simulink model "RAC"  (R2022b)
settings: Solver=FixedStepAuto  StartTime=0.0  StopTime=50000000  FixedStep=1  RelTol=1e-3
libraries: simulink x50
(part 1 of 2)
settings Model: Creator=sadamu  LastModifiedBy=程一帆
settings OptimizationCC: DefaultParameterBehavior=Inlined  BufferReuse=off  GlobalBufferReuse=off  ExpressionFolding=off  EnableMemcpy=off  PassReuseOutputArgsAs=Individual arguments  NoFixptDivByZeroProtection=on  EfficientFloat2IntCast=on  OptimizeDataStoreBuffers=off  BusAssignmentInplaceUpdate=off  OptimizationLevel=level0  EfficientTunableParamExpr=on
settings DebuggingCC: ParameterTunabilityLossMsg=error  AllowSymbolicDim=off
settings SFSimCC: MATLABDynamicMemAlloc=off
settings RTWCC: Description=Embedded Coder  SystemTargetFile=ert.tlc  GenCodeOnly=on  TemplateMakefile=ert_default_tmf
settings CodeAppCC: GenerateComments=off  IgnoreCustomStorageClasses=off  OperatorAnnotations=on  SimulinkDataObjDesc=on  SFDataObjDesc=on  SimulinkBlockComments=off
settings ERTTargetCC: TargetLangStandard=C99 (ISO)  GenerateSampleERTMain=on  CodeInterfacePackaging=Reusable function  InlinedParameterPlacement=NonHierarchical  ERTCustomFileTemplate=example_file_process.tlc
settings ConfigComp: CovMetricSettings=dcmwe  DVMaxProcessTime=3600  DVTestSuiteOptimization=Auto  DVDetectOutOfBounds=on  DVModelReferenceHarness=on

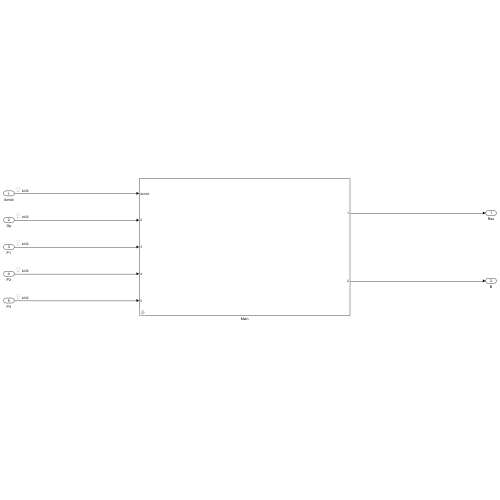
[thumbnail: Simulink's stored preview of the top-level diagram]
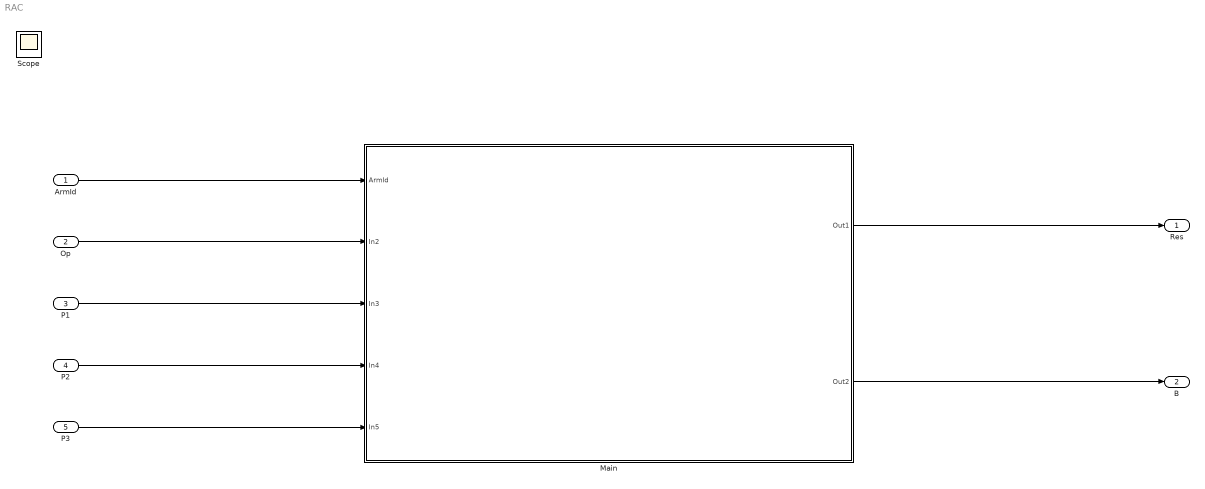
== system RAC ==
  ArmId : Inport  OutDataTypeStr=int32
  Op : Inport  Port=2  OutDataTypeStr=int32
  P1 : Inport  Port=3  OutDataTypeStr=int32
  P2 : Inport  Port=4  OutDataTypeStr=int32
  P3 : Inport  Port=5  OutDataTypeStr=int32
  Main : Subsystem  mask{POOL_SIZE=16}
      mask DialogControl ParameterGroupVar Prompt: 参数
  Res : Outport
  B : Outport  Port=2
  Scope : Scope
  wires:
  ArmId/1 -> Main/1(ArmId)
  Op/1 -> Main/2(In2)
  P1/1 -> Main/3(In3)
  P2/1 -> Main/4(In4)
  P3/1 -> Main/5(In5)
  Main/1(Out1) -> Res/1
  Main/2(Out2) -> B/1

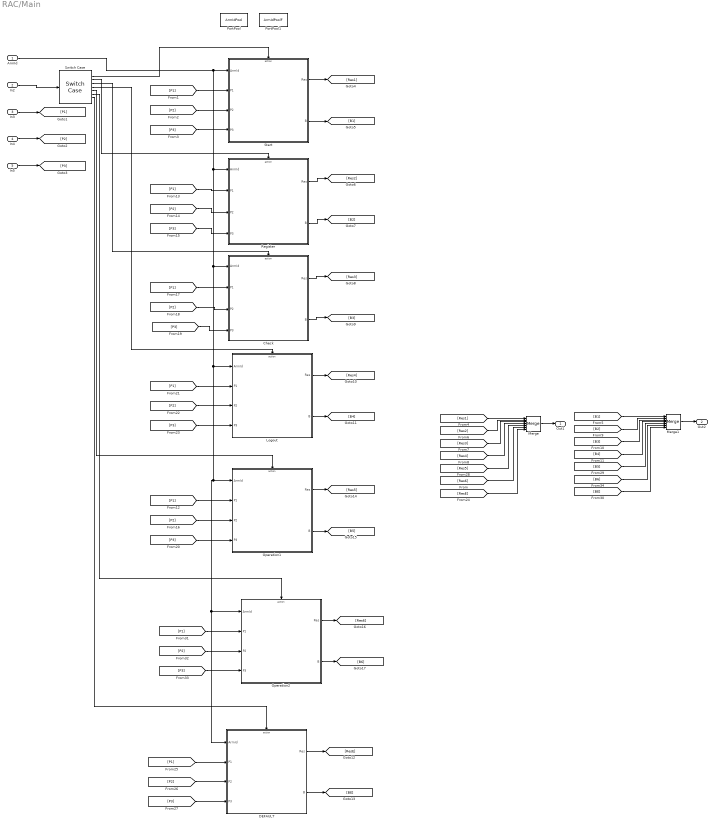
== system RAC/Main ==
  ArmId : Inport
  In2 : Inport  Port=2
  In3 : Inport  Port=3
  In4 : Inport  Port=4
  In5 : Inport  Port=5
  Check : Subsystem  TreatAsAtomicUnit=on
  DEFAULT : Subsystem  TreatAsAtomicUnit=on
  Logout : Subsystem  TreatAsAtomicUnit=on
  Merge : Merge  Inputs=7
  Merge1 : Merge  Inputs=7
  Operation1 : Subsystem  TreatAsAtomicUnit=on
  Operation2 : Subsystem  TreatAsAtomicUnit=on
  PortPool : DataStoreMemory  DataStoreName=ArmIdPool  WriteAfterWriteMsg=warning  ShowAdditionalParam=off  OutDataTypeStr=int32  Dimensions=POOL_SIZE
  PortPool1 : DataStoreMemory  DataStoreName=ArmIdPoolF  WriteAfterWriteMsg=warning  ShowAdditionalParam=off  OutDataTypeStr=int32  Dimensions=POOL_SIZE
  Register : Subsystem  TreatAsAtomicUnit=on
  Start : Subsystem  TreatAsAtomicUnit=on
  Switch Case : SwitchCase  CaseConditions={10001, 10002, 10004, 10008, 10016, 10032}
  Out1 : Outport
  Out2 : Outport  Port=2
  wires:
  DEFAULT/1(Res) -> [ResE]
  Start/1(Res) -> [Res1]
  In2/1 -> Switch Case/1
  [P3] -> Logout/4(P3)
  Check/1(Res) -> [Res3]
  [B4] -> Merge1/4
  [Res1] -> Merge/1
  [B1] -> Merge1/1
  Logout/2(B) -> [B4]
  Check/2(B) -> [B3]
  Start/2(B) -> [B1]
  [Res3] -> Merge/3
  [P3] -> Register/4(P3)
  [P1] -> Start/2(P1)
  [Res5] -> Merge/5
  [Res2] -> Merge/2
  [Res4] -> Merge/4
  [P2] -> Register/3(P2)
  [B2] -> Merge1/2
  [P3] -> DEFAULT/4(P3)
  Register/1(Res) -> [Res2]
  [P1] -> Register/2(P1)
  [P2] -> Start/3(P2)
  [B3] -> Merge1/3
  [P2] -> DEFAULT/3(P2)
  Switch Case/2 -> Register/Action
  In4/1 -> [P2]
  Switch Case/7 -> DEFAULT/Action
  Register/2(B) -> [B2]
  Switch Case/4 -> Logout/Action
  [P2] -> Check/3(P2)
  [B5] -> Merge1/5
  In5/1 -> [P3]
  [P3] -> Start/4(P3)
  [P1] -> DEFAULT/2(P1)
  [P2] -> Logout/3(P2)
  DEFAULT/2(B) -> [BE]
  Switch Case/3 -> Check/Action
  [P1] -> Check/2(P1)
  [P3] -> Check/4(P3)
  Logout/1(Res) -> [Res4]
  Switch Case/1 -> Start/Action
  Merge1/1 -> Out2/1
  [P1] -> Logout/2(P1)
  In3/1 -> [P1]
  Merge/1 -> Out1/1
  [P1] -> Operation1/2(P1)
  [P2] -> Operation1/3(P2)
  Operation1/1(Res) -> [Res5]
  Operation1/2(B) -> [B5]
  [P3] -> Operation1/4(P3)
  Switch Case/5 -> Operation1/Action
  Operation2/1(Res) -> [Res6]
  [P1] -> Operation2/2(P1)
  Operation2/2(B) -> [B6]
  [P3] -> Operation2/4(P3)
  ArmId/1 -> Operation1/1(ArmId), Operation2/1(ArmId), DEFAULT/1(ArmId), Logout/1(ArmId), Check/1(ArmId), Register/1(ArmId), Start/1(ArmId)
  [P2] -> Operation2/3(P2)
  Switch Case/6 -> Operation2/Action
  [B6] -> Merge1/6
  [BE] -> Merge1/7
  [Res6] -> Merge/6
  [ResE] -> Merge/7

== system RAC/Main/Check ==
  ArmId : Inport
  P1 : Inport  Port=2
  P2 : Inport  Port=3
  P3 : Inport  Port=4
  Action Port : ActionPort  ActionPortLabel=case [ 10004 ]:
  Compare To Constant : simulink/Logic and Bit Operations/Compare To Constant  relop===  const=0  OutDataTypeStr=boolean
  Error : Subsystem  TreatAsAtomicUnit=on
  Handle : Subsystem  TreatAsAtomicUnit=on
  If : If  IfExpression=u1 ~= 0
  Merge : Merge
  Merge1 : Merge
  Res : Outport
  B : Outport  Port=2
  wires:
  P1/1 -> Handle/2(P1)
  P2/1 -> Handle/3(P2)
  P3/1 -> Handle/4(P3)
  Merge/1 -> Res/1
  Error/2(B) -> Merge1/1
  If/1 -> Error/Action
  If/2 -> Handle/Action
  Merge1/1 -> B/1
  ArmId/1 -> Handle/1(ArmId), Compare To Constant/1
  Error/1(Res) -> Merge/1
  Handle/2(B) -> Merge1/2
  Handle/1(Res) -> Merge/2
  Compare To Constant/1 -> If/1

== system RAC/Main/DEFAULT ==
  ArmId : Inport
  P1 : Inport  Port=2
  P2 : Inport  Port=3
  P3 : Inport  Port=4
  Action Port : ActionPort  ActionPortLabel=default:
  Constant : Constant  Value=-2  OutDataTypeStr=int32
  Constant1 : Constant  Value=0  OutDataTypeStr=int32
  Terminator{,1..3} (4 alike) : Terminator
  Res : Outport
  B : Outport  Port=2
  wires:
  Constant/1 -> Res/1
  ArmId/1 -> Terminator/1
  P1/1 -> Terminator1/1
  P2/1 -> Terminator2/1
  P3/1 -> Terminator3/1
  Constant1/1 -> B/1

== system RAC/Main/Logout ==
  ArmId : Inport
  P1 : Inport  Port=2
  P2 : Inport  Port=3
  P3 : Inport  Port=4
  Action Port : ActionPort  ActionPortLabel=case [ 10008 ]:
  Compare To Constant : simulink/Logic and Bit Operations/Compare To Constant  relop===  const=0  OutDataTypeStr=boolean
  Error : Subsystem  TreatAsAtomicUnit=on
  Handle : Subsystem  TreatAsAtomicUnit=on
  If : If  IfExpression=u1 ~= 0
  Merge : Merge
  Merge1 : Merge
  Res : Outport
  B : Outport  Port=2
  wires:
  ArmId/1 -> Handle/1(ArmId), Compare To Constant/1
  Compare To Constant/1 -> If/1
  P2/1 -> Handle/3(P2)
  Error/2(B) -> Merge1/1
  P1/1 -> Handle/2(P1)
  Handle/1(Res) -> Merge/2
  Merge1/1 -> B/1
  Error/1(Res) -> Merge/1
  Merge/1 -> Res/1
  If/1 -> Error/Action
  If/2 -> Handle/Action
  P3/1 -> Handle/4(P3)
  Handle/2(B) -> Merge1/2

== system RAC/Main/Operation1 ==
  ArmId : Inport
  P1 : Inport  Port=2
  P2 : Inport  Port=3
  P3 : Inport  Port=4
  Action Port : ActionPort  ActionPortLabel=case [ 10016 ]:
  Compare To Constant : simulink/Logic and Bit Operations/Compare To Constant  relop===  const=0  OutDataTypeStr=boolean
  Error : Subsystem  TreatAsAtomicUnit=on
  Handle : Subsystem  TreatAsAtomicUnit=on
  If : If  IfExpression=u1 ~= 0
  Merge : Merge
  Merge1 : Merge
  Res : Outport
  B : Outport  Port=2
  wires:
  ArmId/1 -> Handle/1(ArmId), Compare To Constant/1
  Compare To Constant/1 -> If/1
  P2/1 -> Handle/3(P2)
  Error/2(B) -> Merge1/1
  P1/1 -> Handle/2(P1)
  Handle/1(Res) -> Merge/2
  Merge1/1 -> B/1
  Error/1(Res) -> Merge/1
  Merge/1 -> Res/1
  If/1 -> Error/Action
  If/2 -> Handle/Action
  P3/1 -> Handle/4(P3)
  Handle/2(B) -> Merge1/2

== system RAC/Main/Operation2 ==
  ArmId : Inport
  P1 : Inport  Port=2
  P2 : Inport  Port=3
  P3 : Inport  Port=4
  Action Port : ActionPort  ActionPortLabel=case [ 10032 ]:
  Compare To Constant : simulink/Logic and Bit Operations/Compare To Constant  relop===  const=0  OutDataTypeStr=boolean
  Error : Subsystem  TreatAsAtomicUnit=on
  Handle : Subsystem  TreatAsAtomicUnit=on
  If : If  IfExpression=u1 ~= 0
  Merge : Merge
  Merge1 : Merge
  Res : Outport
  B : Outport  Port=2
  wires:
  ArmId/1 -> Handle/1(ArmId), Compare To Constant/1
  Compare To Constant/1 -> If/1
  P2/1 -> Handle/3(P2)
  Error/2(B) -> Merge1/1
  P1/1 -> Handle/2(P1)
  Handle/1(Res) -> Merge/2
  Merge1/1 -> B/1
  Error/1(Res) -> Merge/1
  Merge/1 -> Res/1
  If/1 -> Error/Action
  If/2 -> Handle/Action
  P3/1 -> Handle/4(P3)
  Handle/2(B) -> Merge1/2

== system RAC/Main/Register ==
  ArmId : Inport
  P1 : Inport  Port=2
  P2 : Inport  Port=3
  P3 : Inport  Port=4
  Action Port : ActionPort  ActionPortLabel=case [ 10002 ]:
  Compare To Constant : simulink/Logic and Bit Operations/Compare To Constant  relop===  const=0  OutDataTypeStr=boolean
  Error : Subsystem  TreatAsAtomicUnit=on
  Handle : Subsystem  TreatAsAtomicUnit=on
  If : If  IfExpression=u1 ~= 0
  Merge : Merge
  Merge1 : Merge
  Res : Outport
  B : Outport  Port=2
  wires:
  P1/1 -> Handle/2(P1)
  P2/1 -> Handle/3(P2)
  P3/1 -> Handle/4(P3)
  Merge/1 -> Res/1
  Error/2(B) -> Merge1/1
  If/1 -> Error/Action
  If/2 -> Handle/Action
  Merge1/1 -> B/1
  ArmId/1 -> Handle/1(ArmId), Compare To Constant/1
  Error/1(Res) -> Merge/1
  Handle/2(B) -> Merge1/2
  Handle/1(Res) -> Merge/2
  Compare To Constant/1 -> If/1

== system RAC/Main/Start ==
  ArmId : Inport
  P1 : Inport  Port=2
  P2 : Inport  Port=3
  P3 : Inport  Port=4
  Action Port : ActionPort  ActionPortLabel=case [ 10001 ]:
  Compare To Constant : simulink/Logic and Bit Operations/Compare To Constant  relop===  const=0  OutDataTypeStr=boolean
  Error : Subsystem  TreatAsAtomicUnit=on
  Handle : Subsystem  TreatAsAtomicUnit=on
  If : If  IfExpression=u1 ~= 0
  Merge : Merge
  Merge1 : Merge
  Res : Outport
  B : Outport  Port=2
  wires:
  ArmId/1 -> Handle/1(ArmId), Compare To Constant/1
  Compare To Constant/1 -> If/1
  If/1 -> Error/Action
  If/2 -> Handle/Action
  Error/1(Res) -> Merge/1
  Handle/1(Res) -> Merge/2
  Merge/1 -> Res/1
  Merge1/1 -> B/1
  Error/2(B) -> Merge1/1
  Handle/2(B) -> Merge1/2
  P1/1 -> Handle/2(P1)
  P2/1 -> Handle/3(P2)
  P3/1 -> Handle/4(P3)

== system RAC/Main/Check/Error ==
  Action Port : ActionPort  ActionPortLabel=if(u1 ~= 0)
  Constant : Constant  Value=-1  OutDataTypeStr=int32
  Constant1 : Constant  Value=0  OutDataTypeStr=int32
  Res : Outport
  B : Outport  Port=2
  wires:
  Constant/1 -> Res/1
  Constant1/1 -> B/1

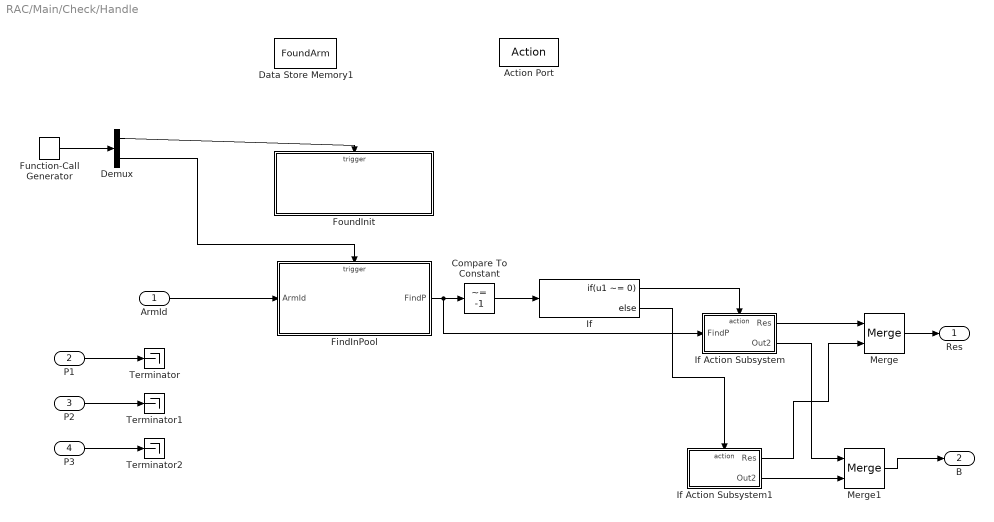
== system RAC/Main/Check/Handle ==
  ArmId : Inport
  P1 : Inport  Port=2
  P2 : Inport  Port=3
  P3 : Inport  Port=4
  Action Port : ActionPort  ActionPortLabel=else
  Compare To Constant : simulink/Logic and Bit Operations/Compare To Constant  relop=~=  const=-1  OutDataTypeStr=boolean
  Data Store Memory1 : DataStoreMemory  DataStoreName=FoundArm  WriteAfterWriteMsg=warning  InitialValue=-1  ShowAdditionalParam=off  OutDataTypeStr=int32
  Demux : Demux  Outputs=2
  FindInPool : Subsystem
  FoundInit : Subsystem
  Function-Call Generator : simulink/Ports & Subsystems/Function-Call Generator  sample_time=1  numberOfIterations=1  DisallowWideOutput=off
  If : If  IfExpression=u1 ~= 0
  If Action Subsystem : Subsystem  TreatAsAtomicUnit=on
  If Action Subsystem1 : Subsystem  TreatAsAtomicUnit=on
  Merge : Merge
  Merge1 : Merge
  Terminator : Terminator
  Terminator1 : Terminator
  Terminator2 : Terminator
  Res : Outport
  B : Outport  Port=2
  wires:
  Function-Call Generator/1 -> Demux/1
  Demux/1 -> FoundInit/Trigger
  Demux/2 -> FindInPool/Trigger
  ArmId/1 -> FindInPool/1(ArmId)
  P1/1 -> Terminator/1
  P2/1 -> Terminator1/1
  P3/1 -> Terminator2/1
  FindInPool/1(FindP) -> If Action Subsystem/1(FindP), Compare To Constant/1
  Compare To Constant/1 -> If/1
  If/1 -> If Action Subsystem/Action
  Merge/1 -> Res/1
  Merge1/1 -> B/1
  If Action Subsystem/1(Res) -> Merge/1
  If Action Subsystem/2(Out2) -> Merge1/1
  If Action Subsystem1/1(Res) -> Merge/2
  If Action Subsystem1/2(Out2) -> Merge1/2
  If/2 -> If Action Subsystem1/Action

== system RAC/Main/Logout/Error ==
  Action Port : ActionPort  ActionPortLabel=if(u1 ~= 0)
  Constant : Constant  Value=-1  OutDataTypeStr=int32
  Constant1 : Constant  Value=0  OutDataTypeStr=int32
  Res : Outport
  B : Outport  Port=2
  wires:
  Constant/1 -> Res/1
  Constant1/1 -> B/1

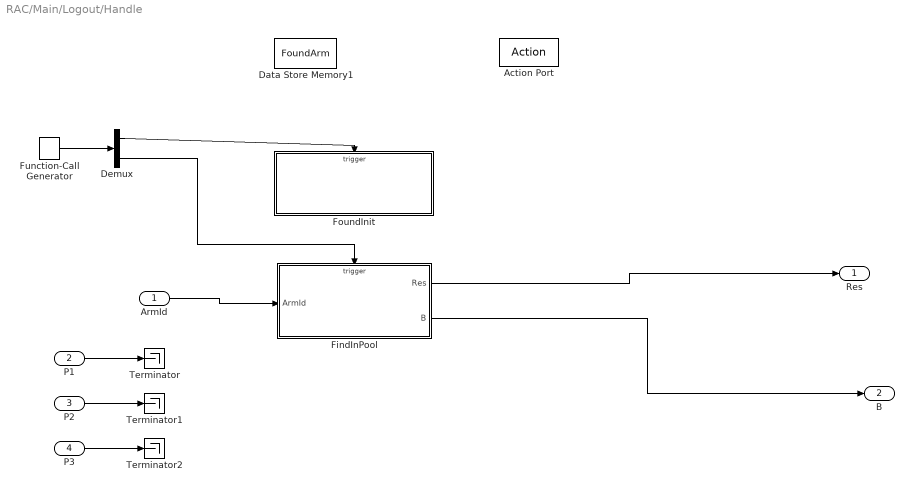
== system RAC/Main/Logout/Handle ==
  ArmId : Inport
  P1 : Inport  Port=2
  P2 : Inport  Port=3
  P3 : Inport  Port=4
  Action Port : ActionPort  ActionPortLabel=else
  Data Store Memory1 : DataStoreMemory  DataStoreName=FoundArm  WriteAfterWriteMsg=warning  InitialValue=-1  ShowAdditionalParam=off  OutDataTypeStr=int32
  Demux : Demux  Outputs=2
  FindInPool : Subsystem
  FoundInit : Subsystem
  Function-Call Generator : simulink/Ports & Subsystems/Function-Call Generator  sample_time=1  numberOfIterations=1  DisallowWideOutput=off
  Terminator : Terminator
  Terminator1 : Terminator
  Terminator2 : Terminator
  Res : Outport
  B : Outport  Port=2
  wires:
  Function-Call Generator/1 -> Demux/1
  Demux/1 -> FoundInit/Trigger
  Demux/2 -> FindInPool/Trigger
  ArmId/1 -> FindInPool/1(ArmId)
  P1/1 -> Terminator/1
  P2/1 -> Terminator1/1
  P3/1 -> Terminator2/1
  FindInPool/1(Res) -> Res/1
  FindInPool/2(B) -> B/1

== system RAC/Main/Operation1/Error ==
  Action Port : ActionPort  ActionPortLabel=if(u1 ~= 0)
  Constant : Constant  Value=-1  OutDataTypeStr=int32
  Constant1 : Constant  Value=0  OutDataTypeStr=int32
  Res : Outport
  B : Outport  Port=2
  wires:
  Constant/1 -> Res/1
  Constant1/1 -> B/1

== system RAC/Main/Operation1/Handle ==
  ArmId : Inport
  P1 : Inport  Port=2
  P2 : Inport  Port=3
  P3 : Inport  Port=4
  Action Port : ActionPort  ActionPortLabel=else
  Data Store Memory1 : DataStoreMemory  DataStoreName=FoundArm  WriteAfterWriteMsg=warning  InitialValue=-1  ShowAdditionalParam=off  OutDataTypeStr=int32
  Demux : Demux  Outputs=2
  FindInPool : Subsystem
  FoundInit : Subsystem
  Function-Call Generator : simulink/Ports & Subsystems/Function-Call Generator  sample_time=1  numberOfIterations=1  DisallowWideOutput=off
  Res : Outport
  B : Outport  Port=2
  wires:
  Function-Call Generator/1 -> Demux/1
  Demux/1 -> FoundInit/Trigger
  Demux/2 -> FindInPool/Trigger
  ArmId/1 -> FindInPool/1(ArmId)
  P1/1 -> FindInPool/2(P1)
  P2/1 -> FindInPool/3(P2)
  P3/1 -> FindInPool/4(P3)
  FindInPool/1(Res) -> Res/1
  FindInPool/2(B) -> B/1

== system RAC/Main/Operation2/Error ==
  Action Port : ActionPort
  Constant : Constant  Value=-1  OutDataTypeStr=int32
  Constant1 : Constant  Value=0  OutDataTypeStr=int32
  Res : Outport
  B : Outport  Port=2
  wires:
  Constant/1 -> Res/1
  Constant1/1 -> B/1

== system RAC/Main/Operation2/Handle ==
  ArmId : Inport
  P1 : Inport  Port=2
  P2 : Inport  Port=3
  P3 : Inport  Port=4
  Action Port : ActionPort
  Data Store Memory1 : DataStoreMemory  DataStoreName=FoundArm  WriteAfterWriteMsg=warning  InitialValue=-1  ShowAdditionalParam=off  OutDataTypeStr=int32
  Demux : Demux  Outputs=2
  FindInPool : Subsystem
  FoundInit : Subsystem
  Function-Call Generator : simulink/Ports & Subsystems/Function-Call Generator  sample_time=1  numberOfIterations=1  DisallowWideOutput=off
  Res : Outport
  B : Outport  Port=2
  wires:
  Function-Call Generator/1 -> Demux/1
  Demux/1 -> FoundInit/Trigger
  Demux/2 -> FindInPool/Trigger
  ArmId/1 -> FindInPool/1(ArmId)
  P1/1 -> FindInPool/2(P1)
  P2/1 -> FindInPool/3(P2)
  P3/1 -> FindInPool/4(P3)
  FindInPool/1(Res) -> Res/1
  FindInPool/2(B) -> B/1

== system RAC/Main/Register/Error ==
  Action Port : ActionPort  ActionPortLabel=if(u1 ~= 0)
  Constant : Constant  Value=-1  OutDataTypeStr=int32
  Constant1 : Constant  Value=0  OutDataTypeStr=int32
  Res : Outport
  B : Outport  Port=2
  wires:
  Constant/1 -> Res/1
  Constant1/1 -> B/1

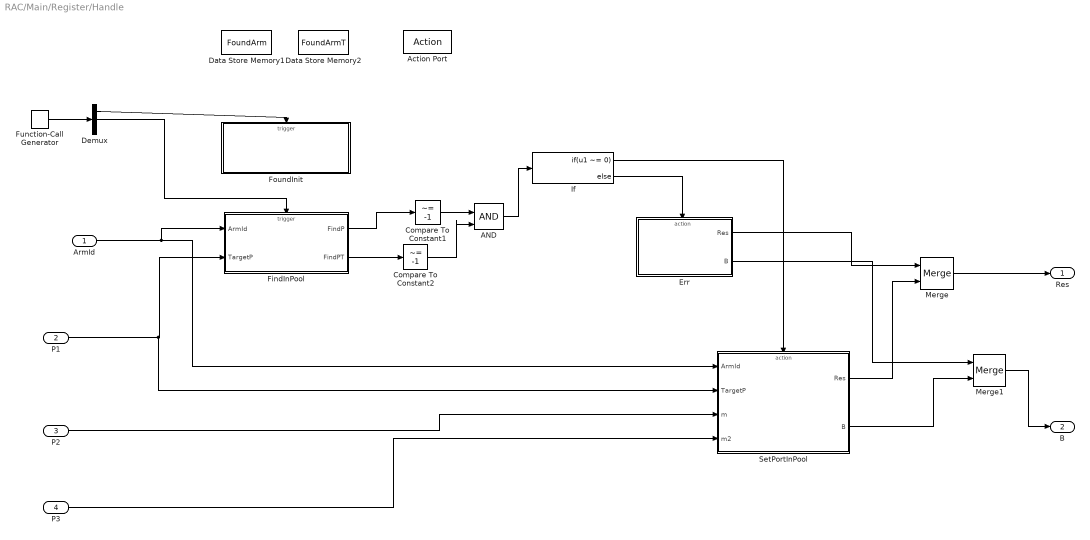
== system RAC/Main/Register/Handle ==
  ArmId : Inport
  P1 : Inport  Port=2
  P2 : Inport  Port=3
  P3 : Inport  Port=4
  Action Port : ActionPort  ActionPortLabel=else
  AND : Logic  IconShape=distinctive  AllPortsSameDT=off  OutDataTypeStr=boolean
  Compare To Constant1 : simulink/Logic and Bit Operations/Compare To Constant  relop=~=  const=-1  OutDataTypeStr=boolean
  Compare To Constant2 : simulink/Logic and Bit Operations/Compare To Constant  relop=~=  const=-1  OutDataTypeStr=boolean
  Data Store Memory1 : DataStoreMemory  DataStoreName=FoundArm  WriteAfterWriteMsg=warning  InitialValue=-1  ShowAdditionalParam=off  OutDataTypeStr=int32
  Data Store Memory2 : DataStoreMemory  DataStoreName=FoundArmT  WriteAfterWriteMsg=warning  InitialValue=-1  ShowAdditionalParam=off  OutDataTypeStr=int32
  Demux : Demux  Outputs=3
  Err : Subsystem  TreatAsAtomicUnit=on
  FindInPool : Subsystem
  FoundInit : Subsystem
  Function-Call Generator : simulink/Ports & Subsystems/Function-Call Generator  sample_time=1  numberOfIterations=1  DisallowWideOutput=off
  If : If  IfExpression=u1 ~= 0
  Merge : Merge
  Merge1 : Merge
  SetPortInPool : Subsystem  TreatAsAtomicUnit=on
  Res : Outport
  B : Outport  Port=2
  wires:
  Function-Call Generator/1 -> Demux/1
  Demux/1 -> FoundInit/Trigger
  Demux/2 -> FindInPool/Trigger
  ArmId/1 -> SetPortInPool/1(ArmId), FindInPool/1(ArmId)
  If/1 -> SetPortInPool/Action
  Merge/1 -> Res/1
  SetPortInPool/2(B) -> Merge1/2
  P3/1 -> SetPortInPool/4(m2)
  FindInPool/1(FindP) -> Compare To Constant1/1
  P1/1 -> SetPortInPool/2(TargetP), FindInPool/2(TargetP)
  FindInPool/2(FindPT) -> Compare To Constant2/1
  Compare To Constant1/1 -> AND/1
  Compare To Constant2/1 -> AND/2
  AND/1 -> If/1
  If/2 -> Err/Action
  SetPortInPool/1(Res) -> Merge/2
  Err/1(Res) -> Merge/1
  P2/1 -> SetPortInPool/3(m)
  Err/2(B) -> Merge1/1
  Merge1/1 -> B/1

== system RAC/Main/Start/Error ==
  Action Port : ActionPort  ActionPortLabel=if(u1 ~= 0)
  Constant : Constant  Value=-1  OutDataTypeStr=int32
  Constant1 : Constant  Value=0  OutDataTypeStr=int32
  Res : Outport
  B : Outport  Port=2
  wires:
  Constant/1 -> Res/1
  Constant1/1 -> B/1

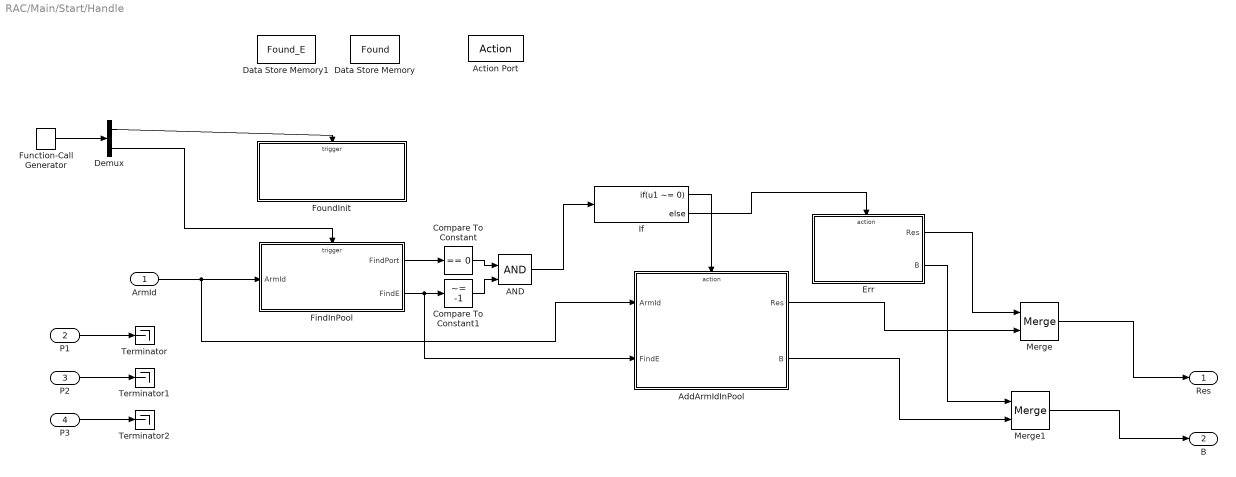
== system RAC/Main/Start/Handle ==
  ArmId : Inport
  P1 : Inport  Port=2
  P2 : Inport  Port=3
  P3 : Inport  Port=4
  Action Port : ActionPort  ActionPortLabel=else
  AND : Logic  IconShape=distinctive  AllPortsSameDT=off  OutDataTypeStr=boolean
  AddArmIdInPool : Subsystem  TreatAsAtomicUnit=on
  Compare To Constant : simulink/Logic and Bit Operations/Compare To Constant  relop===  const=0  OutDataTypeStr=boolean
  Compare To Constant1 : simulink/Logic and Bit Operations/Compare To Constant  relop=~=  const=-1  OutDataTypeStr=boolean
  Data Store Memory : DataStoreMemory  DataStoreName=Found  WriteAfterWriteMsg=warning  ShowAdditionalParam=off  OutDataTypeStr=int8
  Data Store Memory1 : DataStoreMemory  DataStoreName=Found_E  WriteAfterWriteMsg=warning  InitialValue=-1  ShowAdditionalParam=off  OutDataTypeStr=int32
  Demux : Demux  Outputs=2
  Err : Subsystem  TreatAsAtomicUnit=on
  FindInPool : Subsystem
  FoundInit : Subsystem
  Function-Call Generator : simulink/Ports & Subsystems/Function-Call Generator  sample_time=1  numberOfIterations=1  DisallowWideOutput=off
  If : If  IfExpression=u1 ~= 0
  Merge : Merge
  Merge1 : Merge
  Terminator : Terminator
  Terminator1 : Terminator
  Terminator2 : Terminator
  Res : Outport
  B : Outport  Port=2
  wires:
  Function-Call Generator/1 -> Demux/1
  Demux/1 -> FoundInit/Trigger
  Demux/2 -> FindInPool/Trigger
  ArmId/1 -> FindInPool/1(ArmId), AddArmIdInPool/1(ArmId)
  AND/1 -> If/1
  Merge/1 -> Res/1
  Err/1(Res) -> Merge/1
  AddArmIdInPool/1(Res) -> Merge/2
  AddArmIdInPool/2(B) -> Merge1/2
  P1/1 -> Terminator/1
  P2/1 -> Terminator1/1
  P3/1 -> Terminator2/1
  FindInPool/1(FindPort) -> Compare To Constant/1
  FindInPool/2(FindE) -> AddArmIdInPool/2(FindE), Compare To Constant1/1
  Compare To Constant/1 -> AND/1
  Compare To Constant1/1 -> AND/2
  If/2 -> Err/Action
  If/1 -> AddArmIdInPool/Action
  Err/2(B) -> Merge1/1
  Merge1/1 -> B/1

== system RAC/Main/Check/Handle/FindInPool ==
  ArmId : Inport
  function : TriggerPort  TriggerType=function-call  VariantControl=(inherit)
  FindArmIdInPool : Subsystem  TreatAsAtomicUnit=on
  FindP : Outport
  wires:
  ArmId/1 -> FindArmIdInPool/1(ArmId)
  FindArmIdInPool/1(Out1) -> FindP/1

== system RAC/Main/Check/Handle/FoundInit ==
  function : TriggerPort  TriggerType=function-call  VariantControl=(inherit)
  Constant1 : Constant  Value=-1  OutDataTypeStr=int32
  Data Store Write1 : DataStoreWrite  DataStoreName=FoundArm  IndexOptions=Index vector (dialog)  Indices=1  OutputSizes=1
  wires:
  Constant1/1 -> Data Store Write1/1

== system RAC/Main/Check/Handle/If Action Subsystem ==
  FindP : Inport
  Action Port : ActionPort  ActionPortLabel=if(u1 ~= 0)
  Constant : Constant  OutDataTypeStr=int32
  Res : Outport
  Out2 : Outport  Port=2
  wires:
  FindP/1 -> Res/1
  Constant/1 -> Out2/1

== system RAC/Main/Check/Handle/If Action Subsystem1 ==
  Action Port : ActionPort  ActionPortLabel=else
  Constant : Constant  Value=-1  OutDataTypeStr=int32
  Constant1 : Constant  Value=-1  OutDataTypeStr=int32
  Res : Outport
  Out2 : Outport  Port=2
  wires:
  Constant/1 -> Out2/1
  Constant1/1 -> Res/1

== system RAC/Main/Logout/Handle/FindInPool ==
  ArmId : Inport
  function : TriggerPort  TriggerType=function-call  VariantControl=(inherit)
  Compare To Constant1 : simulink/Logic and Bit Operations/Compare To Constant  relop===  const=-1  OutDataTypeStr=uint8
  Err : Subsystem  TreatAsAtomicUnit=on
  FindArmIdInPool : Subsystem  TreatAsAtomicUnit=on
  If : If  IfExpression=u1 ~= 0
  Merge : Merge
  Merge1 : Merge
  SetArmIdInPool : Subsystem  TreatAsAtomicUnit=on
  Res : Outport
  B : Outport  Port=2
  wires:
  SetArmIdInPool/2(B) -> Merge1/2
  If/1 -> Err/Action
  ArmId/1 -> SetArmIdInPool/1(ArmId), FindArmIdInPool/1(ArmId)
  FindArmIdInPool/1(Out1) -> Compare To Constant1/1
  Err/1(Res) -> Merge/1
  If/2 -> SetArmIdInPool/Action
  Compare To Constant1/1 -> If/1
  Merge/1 -> Res/1
  SetArmIdInPool/1(Res) -> Merge/2
  Err/2(B) -> Merge1/1
  Merge1/1 -> B/1

== system RAC/Main/Logout/Handle/FoundInit ==
  function : TriggerPort  TriggerType=function-call  VariantControl=(inherit)
  Constant1 : Constant  Value=-1  OutDataTypeStr=int32
  Data Store Write1 : DataStoreWrite  DataStoreName=FoundArm  IndexOptions=Index vector (dialog)  Indices=1  OutputSizes=1
  wires:
  Constant1/1 -> Data Store Write1/1

== system RAC/Main/Operation1/Handle/FindInPool ==
  ArmId : Inport
  P1 : Inport  Port=2
  P2 : Inport  Port=3
  P3 : Inport  Port=4
  function : TriggerPort  TriggerType=function-call  VariantControl=(inherit)
  Compare To Constant1 : simulink/Logic and Bit Operations/Compare To Constant  relop===  const=-1  OutDataTypeStr=uint8
  Err : Subsystem  TreatAsAtomicUnit=on
  FindArmIdInPool : Subsystem  TreatAsAtomicUnit=on
  If : If  IfExpression=u1 ~= 0
  Merge : Merge
  Merge1 : Merge
  SetArmIdInPool : Subsystem  TreatAsAtomicUnit=on
  Res : Outport
  B : Outport  Port=2
  wires:
  SetArmIdInPool/2(B) -> Merge1/2
  If/1 -> Err/Action
  ArmId/1 -> SetArmIdInPool/1(ArmId), FindArmIdInPool/1(ArmId)
  FindArmIdInPool/1(Out1) -> Compare To Constant1/1
  Err/1(Res) -> Merge/1
  If/2 -> SetArmIdInPool/Action
  Compare To Constant1/1 -> If/1
  Merge/1 -> Res/1
  SetArmIdInPool/1(Res) -> Merge/2
  P1/1 -> SetArmIdInPool/2(P1)
  P2/1 -> SetArmIdInPool/3(P2)
  P3/1 -> SetArmIdInPool/4(P3)
  Err/2(B) -> Merge1/1
  Merge1/1 -> B/1

== system RAC/Main/Operation1/Handle/FoundInit ==
  function : TriggerPort  TriggerType=function-call  VariantControl=(inherit)
  Constant1 : Constant  Value=-1  OutDataTypeStr=int32
  Data Store Write1 : DataStoreWrite  DataStoreName=FoundArm  IndexOptions=Index vector (dialog)  Indices=1  OutputSizes=1
  wires:
  Constant1/1 -> Data Store Write1/1

== system RAC/Main/Operation2/Handle/FindInPool ==
  ArmId : Inport
  P1 : Inport  Port=2
  P2 : Inport  Port=3
  P3 : Inport  Port=4
  function : TriggerPort  TriggerType=function-call  VariantControl=(inherit)
  Compare To Constant1 : simulink/Logic and Bit Operations/Compare To Constant  relop===  const=-1  OutDataTypeStr=uint8
  Err : Subsystem  TreatAsAtomicUnit=on
  FindArmIdInPool : Subsystem  TreatAsAtomicUnit=on
  If : If  IfExpression=u1 ~= 0
  Merge : Merge
  Merge1 : Merge
  SetArmIdInPool : Subsystem  TreatAsAtomicUnit=on
  Res : Outport
  B : Outport  Port=2
  wires:
  SetArmIdInPool/2(B) -> Merge1/2
  If/1 -> Err/Action
  ArmId/1 -> SetArmIdInPool/1(ArmId), FindArmIdInPool/1(ArmId)
  FindArmIdInPool/1(Out1) -> Compare To Constant1/1
  Err/1(Res) -> Merge/1
  If/2 -> SetArmIdInPool/Action
  Compare To Constant1/1 -> If/1
  Merge/1 -> Res/1
  SetArmIdInPool/1(Res) -> Merge/2
  P1/1 -> SetArmIdInPool/2(P1)
  P2/1 -> SetArmIdInPool/3(P2)
  P3/1 -> SetArmIdInPool/4(P3)
  Err/2(B) -> Merge1/1
  Merge1/1 -> B/1

== system RAC/Main/Operation2/Handle/FoundInit ==
  function : TriggerPort  TriggerType=function-call  VariantControl=(inherit)
  Constant1 : Constant  Value=-1  OutDataTypeStr=int32
  Data Store Write1 : DataStoreWrite  DataStoreName=FoundArm  IndexOptions=Index vector (dialog)  Indices=1  OutputSizes=1
  wires:
  Constant1/1 -> Data Store Write1/1

== system RAC/Main/Register/Handle/Err ==
  Action Port : ActionPort  ActionPortLabel=else
  Constant : Constant  Value=-3  OutDataTypeStr=int32
  Constant1 : Constant  OutDataTypeStr=int32
  Res : Outport
  B : Outport  Port=2
  wires:
  Constant/1 -> Res/1
  Constant1/1 -> B/1

== system RAC/Main/Register/Handle/FindInPool ==
  ArmId : Inport
  TargetP : Inport  Port=2
  function : TriggerPort  TriggerType=function-call  VariantControl=(inherit)
  FindArmIdInPool : Subsystem  TreatAsAtomicUnit=on
  FindArmIdTInPool : Subsystem  TreatAsAtomicUnit=on
  FindP : Outport
  FindPT : Outport  Port=2
  wires:
  ArmId/1 -> FindArmIdInPool/1(ArmId)
  FindArmIdInPool/1(Out1) -> FindP/1
  TargetP/1 -> FindArmIdTInPool/1(ArmId)
  FindArmIdTInPool/1(FindPT) -> FindPT/1

== system RAC/Main/Register/Handle/FoundInit ==
  function : TriggerPort  TriggerType=function-call  VariantControl=(inherit)
  Constant1 : Constant  Value=-1  OutDataTypeStr=int32
  Constant2 : Constant  Value=-1  OutDataTypeStr=int32
  Data Store Write1 : DataStoreWrite  DataStoreName=FoundArm  IndexOptions=Index vector (dialog)  Indices=1  OutputSizes=1
  Data Store Write2 : DataStoreWrite  DataStoreName=FoundArmT  IndexOptions=Index vector (dialog)  Indices=1  OutputSizes=1
  wires:
  Constant1/1 -> Data Store Write1/1
  Constant2/1 -> Data Store Write2/1

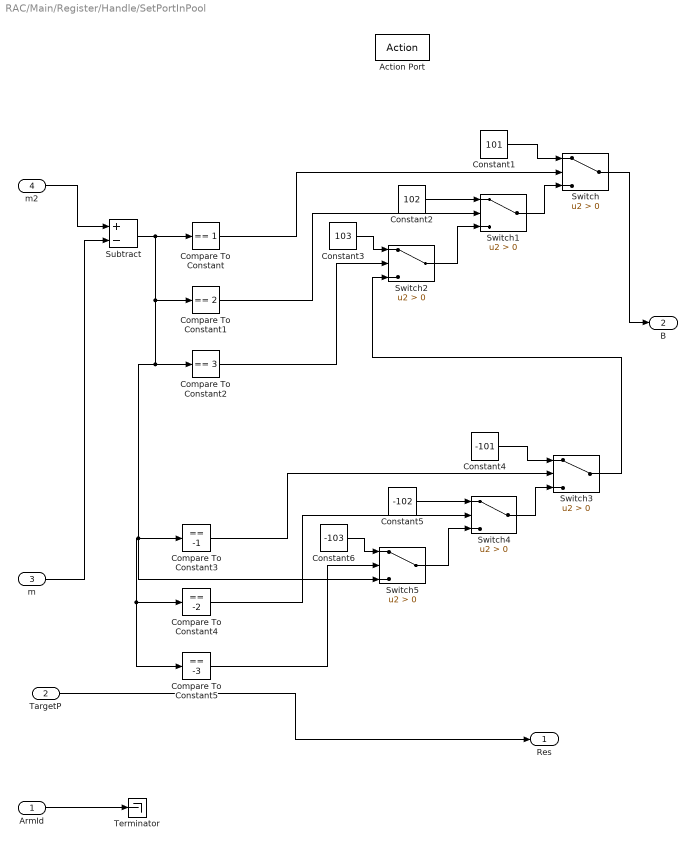
== system RAC/Main/Register/Handle/SetPortInPool ==
  ArmId : Inport
  TargetP : Inport  Port=2
  m : Inport  Port=3
  m2 : Inport  Port=4
  Action Port : ActionPort  ActionPortLabel=if(u1 ~= 0)
  Compare To Constant : simulink/Logic and Bit Operations/Compare To Constant  relop===  const=1  OutDataTypeStr=boolean
  Compare To Constant1 : simulink/Logic and Bit Operations/Compare To Constant  relop===  const=2  OutDataTypeStr=boolean
  Compare To Constant2 : simulink/Logic and Bit Operations/Compare To Constant  relop===  const=3  OutDataTypeStr=boolean
  Compare To Constant3 : simulink/Logic and Bit Operations/Compare To Constant  relop===  const=-1  OutDataTypeStr=boolean
  Compare To Constant4 : simulink/Logic and Bit Operations/Compare To Constant  relop===  const=-2  OutDataTypeStr=boolean
  Compare To Constant5 : simulink/Logic and Bit Operations/Compare To Constant  relop===  const=-3  OutDataTypeStr=boolean
  Constant1 : Constant  Value=101  OutDataTypeStr=int32
  Constant2 : Constant  Value=102  OutDataTypeStr=int32
  Constant3 : Constant  Value=103  OutDataTypeStr=int32
  Constant4 : Constant  Value=-101  OutDataTypeStr=int32
  Constant5 : Constant  Value=-102  OutDataTypeStr=int32
  Constant6 : Constant  Value=-103  OutDataTypeStr=int32
  Subtract : Sum  Inputs=+-
  Switch{,1..5} (6 alike) : Switch  Criteria=u2 > Threshold  SaturateOnIntegerOverflow=off  InputSameDT=off
  Terminator : Terminator
  Res : Outport
  B : Outport  Port=2
  wires:
  Compare To Constant/1 -> Switch/2
  Constant1/1 -> Switch/1
  Compare To Constant1/1 -> Switch1/2
  Constant2/1 -> Switch1/1
  Switch1/1 -> Switch/3
  Constant3/1 -> Switch2/1
  Switch2/1 -> Switch1/3
  Compare To Constant2/1 -> Switch2/2
  Constant4/1 -> Switch3/1
  Constant6/1 -> Switch5/1
  Constant5/1 -> Switch4/1
  Compare To Constant4/1 -> Switch4/2
  Compare To Constant5/1 -> Switch5/2
  Switch4/1 -> Switch3/3
  Subtract/1 -> Switch5/3, Compare To Constant5/1, Compare To Constant4/1, Compare To Constant3/1, Compare To Constant2/1, Compare To Constant1/1, Compare To Constant/1
  Compare To Constant3/1 -> Switch3/2
  Switch5/1 -> Switch4/3
  Switch3/1 -> Switch2/3
  Switch/1 -> B/1
  m/1 -> Subtract/2
  TargetP/1 -> Res/1
  m2/1 -> Subtract/1
  ArmId/1 -> Terminator/1

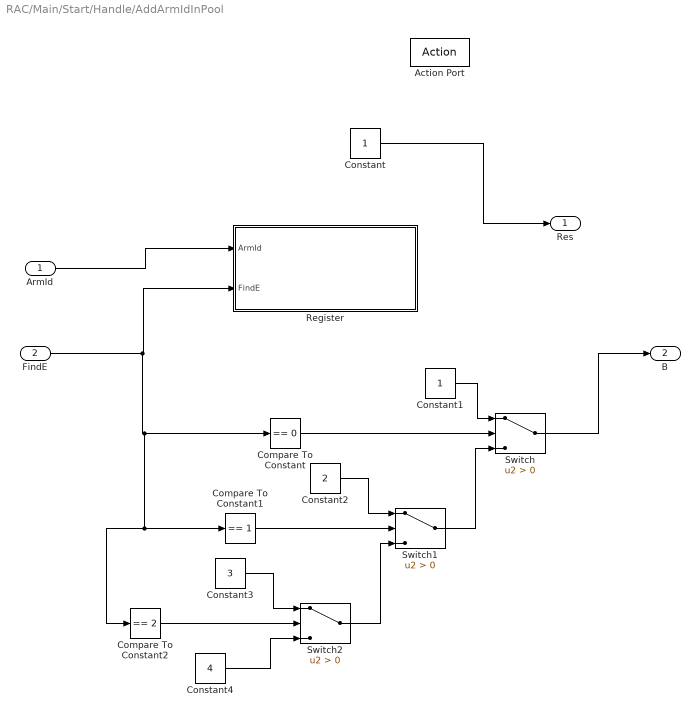
== system RAC/Main/Start/Handle/AddArmIdInPool ==
  ArmId : Inport
  FindE : Inport  Port=2
  Action Port : ActionPort  ActionPortLabel=if(u1 ~= 0)
  Compare To Constant : simulink/Logic and Bit Operations/Compare To Constant  relop===  const=0  OutDataTypeStr=boolean
  Compare To Constant1 : simulink/Logic and Bit Operations/Compare To Constant  relop===  const=1  OutDataTypeStr=boolean
  Compare To Constant2 : simulink/Logic and Bit Operations/Compare To Constant  relop===  const=2  OutDataTypeStr=boolean
  Constant : Constant  OutDataTypeStr=int32
  Constant1 : Constant  OutDataTypeStr=int32
  Constant2 : Constant  Value=2  OutDataTypeStr=int32
  Constant3 : Constant  Value=3  OutDataTypeStr=int32
  Constant4 : Constant  Value=4  OutDataTypeStr=int32
  Register : Subsystem  TreatAsAtomicUnit=on
  Switch : Switch  Criteria=u2 > Threshold  SaturateOnIntegerOverflow=off  InputSameDT=off
  Switch1 : Switch  Criteria=u2 > Threshold  SaturateOnIntegerOverflow=off  InputSameDT=off
  Switch2 : Switch  Criteria=u2 > Threshold  SaturateOnIntegerOverflow=off  InputSameDT=off
  Res : Outport
  B : Outport  Port=2
  wires:
  ArmId/1 -> Register/1(ArmId)
  FindE/1 -> Compare To Constant2/1, Compare To Constant1/1, Compare To Constant/1, Register/2(FindE)
  Constant/1 -> Res/1
  Compare To Constant/1 -> Switch/2
  Constant1/1 -> Switch/1
  Constant2/1 -> Switch1/1
  Compare To Constant1/1 -> Switch1/2
  Switch1/1 -> Switch/3
  Compare To Constant2/1 -> Switch2/2
  Switch2/1 -> Switch1/3
  Constant3/1 -> Switch2/1
  Constant4/1 -> Switch2/3
  Switch/1 -> B/1

== system RAC/Main/Start/Handle/Err ==
  Action Port : ActionPort  ActionPortLabel=else
  Constant : Constant  Value=-4  OutDataTypeStr=int32
  Constant1 : Constant  OutDataTypeStr=int32
  Res : Outport
  B : Outport  Port=2
  wires:
  Constant/1 -> Res/1
  Constant1/1 -> B/1

== system RAC/Main/Start/Handle/FindInPool ==
  ArmId : Inport
  function : TriggerPort  TriggerType=function-call  VariantControl=(inherit)
  FindArmIdInPool : Subsystem  TreatAsAtomicUnit=on
  FindEmptyInPool : Subsystem  TreatAsAtomicUnit=on
  FindPort : Outport
  FindE : Outport  Port=2
  wires:
  FindArmIdInPool/1(Out1) -> FindPort/1
  ArmId/1 -> FindArmIdInPool/1(ArmId)
  FindEmptyInPool/1(Out1) -> FindE/1

== system RAC/Main/Start/Handle/FoundInit ==
  function : TriggerPort  TriggerType=function-call  VariantControl=(inherit)
  Constant : Constant  Value=0  OutDataTypeStr=int8
  Constant1 : Constant  Value=-1  OutDataTypeStr=int32
  Data Store Write : DataStoreWrite  DataStoreName=Found  IndexOptions=Index vector (dialog)  Indices=1  OutputSizes=1
  Data Store Write1 : DataStoreWrite  DataStoreName=Found_E  IndexOptions=Index vector (dialog)  Indices=1  OutputSizes=1
  wires:
  Constant/1 -> Data Store Write/1
  Constant1/1 -> Data Store Write1/1

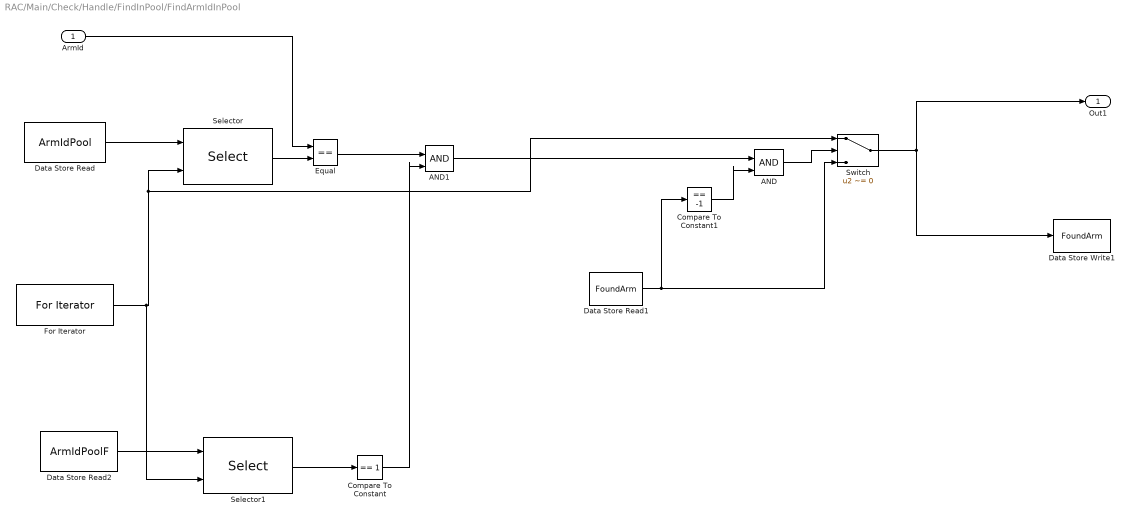
== system RAC/Main/Check/Handle/FindInPool/FindArmIdInPool ==
  ArmId : Inport
  AND : Logic  IconShape=distinctive  AllPortsSameDT=off  OutDataTypeStr=boolean
  AND1 : Logic  IconShape=distinctive  AllPortsSameDT=off  OutDataTypeStr=boolean
  Compare To Constant : simulink/Logic and Bit Operations/Compare To Constant  relop===  const=1  OutDataTypeStr=boolean
  Compare To Constant1 : simulink/Logic and Bit Operations/Compare To Constant  relop===  const=-1  OutDataTypeStr=boolean
  Data Store Read : DataStoreRead  DataStoreName=ArmIdPool  IndexOptions=Index vector (dialog)  Indices=1  OutputSizes=1
  Data Store Read1 : DataStoreRead  DataStoreName=FoundArm  IndexOptions=Index vector (dialog)  Indices=1  OutputSizes=1
  Data Store Read2 : DataStoreRead  DataStoreName=ArmIdPoolF  IndexOptions=Index vector (dialog)  Indices=1  OutputSizes=1
  Data Store Write1 : DataStoreWrite  DataStoreName=FoundArm  IndexOptions=Index vector (dialog)  Indices=1  OutputSizes=1
  Equal : RelationalOperator  Operator===  OutDataTypeStr=boolean  RndMeth=Simplest  InputSameDT=off
  For Iterator : ForIterator  IterationLimit=POOL_SIZE  IndexMode=Zero-based
  Selector : Selector  IndexMode=Zero-based  InputPortWidth=POOL_SIZE  IndexOptions=Index vector (port)  Indices=[1 3]  OutputSizes=1
  Selector1 : Selector  IndexMode=Zero-based  InputPortWidth=POOL_SIZE  IndexOptions=Index vector (port)  Indices=[1 3]  OutputSizes=1
  Switch : Switch  Criteria=u2 ~= 0  SaturateOnIntegerOverflow=off  InputSameDT=off
  Out1 : Outport
  wires:
  Data Store Read/1 -> Selector/1
  Selector/1 -> Equal/2
  Equal/1 -> AND1/1
  Switch/1 -> Data Store Write1/1, Out1/1
  Data Store Read1/1 -> Compare To Constant1/1, Switch/3
  Compare To Constant1/1 -> AND/2
  AND/1 -> Switch/2
  ArmId/1 -> Equal/1
  Compare To Constant/1 -> AND1/2
  Data Store Read2/1 -> Selector1/1
  For Iterator/1 -> Selector1/2, Switch/1, Selector/2
  Selector1/1 -> Compare To Constant/1
  AND1/1 -> AND/1

== system RAC/Main/Logout/Handle/FindInPool/Err ==
  Action Port : ActionPort  ActionPortLabel=if(u1 ~= 0)
  Constant : Constant  Value=-3  OutDataTypeStr=int32
  Constant1 : Constant  OutDataTypeStr=int32
  Res : Outport
  B : Outport  Port=2
  wires:
  Constant/1 -> Res/1
  Constant1/1 -> B/1

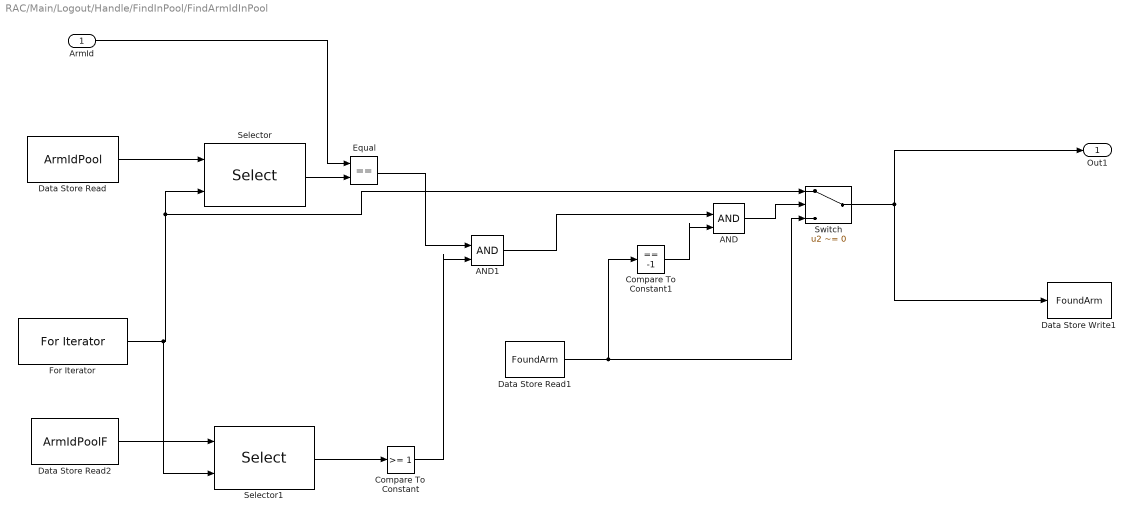
== system RAC/Main/Logout/Handle/FindInPool/FindArmIdInPool ==
  ArmId : Inport
  AND : Logic  IconShape=distinctive  AllPortsSameDT=off  OutDataTypeStr=boolean
  AND1 : Logic  IconShape=distinctive  AllPortsSameDT=off  OutDataTypeStr=boolean
  Compare To Constant : simulink/Logic and Bit Operations/Compare To Constant  relop=>=  const=1  OutDataTypeStr=boolean
  Compare To Constant1 : simulink/Logic and Bit Operations/Compare To Constant  relop===  const=-1  OutDataTypeStr=boolean
  Data Store Read : DataStoreRead  DataStoreName=ArmIdPool  IndexOptions=Index vector (dialog)  Indices=1  OutputSizes=1
  Data Store Read1 : DataStoreRead  DataStoreName=FoundArm  IndexOptions=Index vector (dialog)  Indices=1  OutputSizes=1
  Data Store Read2 : DataStoreRead  DataStoreName=ArmIdPoolF  IndexOptions=Index vector (dialog)  Indices=1  OutputSizes=1
  Data Store Write1 : DataStoreWrite  DataStoreName=FoundArm  IndexOptions=Index vector (dialog)  Indices=1  OutputSizes=1
  Equal : RelationalOperator  Operator===  OutDataTypeStr=boolean  RndMeth=Simplest  InputSameDT=off
  For Iterator : ForIterator  IterationLimit=POOL_SIZE  IndexMode=Zero-based
  Selector : Selector  IndexMode=Zero-based  InputPortWidth=POOL_SIZE  IndexOptions=Index vector (port)  Indices=[1 3]  OutputSizes=1
  Selector1 : Selector  IndexMode=Zero-based  InputPortWidth=POOL_SIZE  IndexOptions=Index vector (port)  Indices=[1 3]  OutputSizes=1
  Switch : Switch  Criteria=u2 ~= 0  SaturateOnIntegerOverflow=off  InputSameDT=off
  Out1 : Outport
  wires:
  Data Store Read/1 -> Selector/1
  Selector/1 -> Equal/2
  Equal/1 -> AND1/1
  Switch/1 -> Data Store Write1/1, Out1/1
  Data Store Read1/1 -> Compare To Constant1/1, Switch/3
  Compare To Constant1/1 -> AND/2
  AND/1 -> Switch/2
  ArmId/1 -> Equal/1
  Compare To Constant/1 -> AND1/2
  Data Store Read2/1 -> Selector1/1
  For Iterator/1 -> Selector1/2, Switch/1, Selector/2
  Selector1/1 -> Compare To Constant/1
  AND1/1 -> AND/1

== system RAC/Main/Logout/Handle/FindInPool/SetArmIdInPool ==
  ArmId : Inport
  Action Port : ActionPort  ActionPortLabel=else
  Constant : Constant  OutDataTypeStr=int32
  LOGOUT : Subsystem  TreatAsAtomicUnit=on
  Res : Outport
  B : Outport  Port=2
  wires:
  ArmId/1 -> Res/1, LOGOUT/1(FindP)
  Constant/1 -> B/1

== system RAC/Main/Operation1/Handle/FindInPool/Err ==
  Action Port : ActionPort  ActionPortLabel=if(u1 ~= 0)
  Constant : Constant  Value=-3  OutDataTypeStr=int32
  Constant1 : Constant  OutDataTypeStr=int32
  Res : Outport
  B : Outport  Port=2
  wires:
  Constant/1 -> Res/1
  Constant1/1 -> B/1

== system RAC/Main/Operation1/Handle/FindInPool/FindArmIdInPool ==
  ArmId : Inport
  AND : Logic  IconShape=distinctive  AllPortsSameDT=off  OutDataTypeStr=boolean
  AND1 : Logic  IconShape=distinctive  AllPortsSameDT=off  OutDataTypeStr=boolean
  Compare To Constant : simulink/Logic and Bit Operations/Compare To Constant  relop=>=  const=1  OutDataTypeStr=boolean
  Compare To Constant1 : simulink/Logic and Bit Operations/Compare To Constant  relop===  const=-1  OutDataTypeStr=boolean
  Data Store Read : DataStoreRead  DataStoreName=ArmIdPool  IndexOptions=Index vector (dialog)  Indices=1  OutputSizes=1
  Data Store Read1 : DataStoreRead  DataStoreName=FoundArm  IndexOptions=Index vector (dialog)  Indices=1  OutputSizes=1
  Data Store Read2 : DataStoreRead  DataStoreName=ArmIdPoolF  IndexOptions=Index vector (dialog)  Indices=1  OutputSizes=1
  Data Store Write1 : DataStoreWrite  DataStoreName=FoundArm  IndexOptions=Index vector (dialog)  Indices=1  OutputSizes=1
  Equal : RelationalOperator  Operator===  OutDataTypeStr=boolean  RndMeth=Simplest  InputSameDT=off
  For Iterator : ForIterator  IterationLimit=POOL_SIZE  IndexMode=Zero-based
  Selector : Selector  IndexMode=Zero-based  InputPortWidth=POOL_SIZE  IndexOptions=Index vector (port)  Indices=[1 3]  OutputSizes=1
  Selector1 : Selector  IndexMode=Zero-based  InputPortWidth=POOL_SIZE  IndexOptions=Index vector (port)  Indices=[1 3]  OutputSizes=1
  Switch : Switch  Criteria=u2 ~= 0  SaturateOnIntegerOverflow=off  InputSameDT=off
  Out1 : Outport
  wires:
  Data Store Read/1 -> Selector/1
  Selector/1 -> Equal/2
  Equal/1 -> AND1/1
  Switch/1 -> Data Store Write1/1, Out1/1
  Data Store Read1/1 -> Compare To Constant1/1, Switch/3
  Compare To Constant1/1 -> AND/2
  AND/1 -> Switch/2
  ArmId/1 -> Equal/1
  Compare To Constant/1 -> AND1/2
  Data Store Read2/1 -> Selector1/1
  For Iterator/1 -> Selector1/2, Switch/1, Selector/2
  Selector1/1 -> Compare To Constant/1
  AND1/1 -> AND/1

== system RAC/Main/Operation1/Handle/FindInPool/SetArmIdInPool ==
  ArmId : Inport
  P1 : Inport  Port=2
  P2 : Inport  Port=3
  P3 : Inport  Port=4
  Action Port : ActionPort  ActionPortLabel=else
  Constant : Constant  OutDataTypeStr=int32
  Operation : Subsystem  TreatAsAtomicUnit=on
  Res : Outport
  B : Outport  Port=2
  wires:
  ArmId/1 -> Res/1, Operation/1(FindP)
  Constant/1 -> B/1
  P1/1 -> Operation/2(P1)
  P2/1 -> Operation/3(P2)
  P3/1 -> Operation/4(P3)

== system RAC/Main/Operation2/Handle/FindInPool/Err ==
  Action Port : ActionPort
  Constant : Constant  Value=-3  OutDataTypeStr=int32
  Constant1 : Constant  OutDataTypeStr=int32
  Res : Outport
  B : Outport  Port=2
  wires:
  Constant/1 -> Res/1
  Constant1/1 -> B/1

== system RAC/Main/Operation2/Handle/FindInPool/FindArmIdInPool ==
  ArmId : Inport
  AND : Logic  IconShape=distinctive  AllPortsSameDT=off  OutDataTypeStr=boolean
  AND1 : Logic  IconShape=distinctive  AllPortsSameDT=off  OutDataTypeStr=boolean
  Compare To Constant : simulink/Logic and Bit Operations/Compare To Constant  relop===  const=5  OutDataTypeStr=boolean
  Compare To Constant1 : simulink/Logic and Bit Operations/Compare To Constant  relop===  const=-1  OutDataTypeStr=boolean
  Data Store Read : DataStoreRead  DataStoreName=ArmIdPool  IndexOptions=Index vector (dialog)  Indices=1  OutputSizes=1
  Data Store Read1 : DataStoreRead  DataStoreName=FoundArm  IndexOptions=Index vector (dialog)  Indices=1  OutputSizes=1
  Data Store Read2 : DataStoreRead  DataStoreName=ArmIdPoolF  IndexOptions=Index vector (dialog)  Indices=1  OutputSizes=1
  Data Store Write1 : DataStoreWrite  DataStoreName=FoundArm  IndexOptions=Index vector (dialog)  Indices=1  OutputSizes=1
  Equal : RelationalOperator  Operator===  OutDataTypeStr=boolean  RndMeth=Simplest  InputSameDT=off
  For Iterator : ForIterator  IterationLimit=POOL_SIZE  IndexMode=Zero-based
  Selector : Selector  IndexMode=Zero-based  InputPortWidth=POOL_SIZE  IndexOptions=Index vector (port)  Indices=[1 3]  OutputSizes=1
  Selector1 : Selector  IndexMode=Zero-based  InputPortWidth=POOL_SIZE  IndexOptions=Index vector (port)  Indices=[1 3]  OutputSizes=1
  Switch : Switch  Criteria=u2 ~= 0  SaturateOnIntegerOverflow=off  InputSameDT=off
  Out1 : Outport
  wires:
  Data Store Read/1 -> Selector/1
  Selector/1 -> Equal/2
  Equal/1 -> AND1/1
  Switch/1 -> Data Store Write1/1, Out1/1
  Data Store Read1/1 -> Compare To Constant1/1, Switch/3
  Compare To Constant1/1 -> AND/2
  AND/1 -> Switch/2
  ArmId/1 -> Equal/1
  Compare To Constant/1 -> AND1/2
  Data Store Read2/1 -> Selector1/1
  For Iterator/1 -> Selector1/2, Switch/1, Selector/2
  Selector1/1 -> Compare To Constant/1
  AND1/1 -> AND/1

== system RAC/Main/Operation2/Handle/FindInPool/SetArmIdInPool ==
  ArmId : Inport
  P1 : Inport  Port=2
  P2 : Inport  Port=3
  P3 : Inport  Port=4
  Action Port : ActionPort
  Constant : Constant  OutDataTypeStr=int32
  Operation : Subsystem  TreatAsAtomicUnit=on
  Res : Outport
  B : Outport  Port=2
  wires:
  ArmId/1 -> Res/1, Operation/1(FindP)
  Constant/1 -> B/1
  P1/1 -> Operation/2(P1)
  P2/1 -> Operation/3(P2)
  P3/1 -> Operation/4(P3)

== system RAC/Main/Register/Handle/FindInPool/FindArmIdInPool ==
  ArmId : Inport
  AND : Logic  IconShape=distinctive  AllPortsSameDT=off  OutDataTypeStr=boolean
  AND1 : Logic  IconShape=distinctive  AllPortsSameDT=off  OutDataTypeStr=boolean
  Compare To Constant : simulink/Logic and Bit Operations/Compare To Constant  relop===  const=1  OutDataTypeStr=boolean
  Compare To Constant1 : simulink/Logic and Bit Operations/Compare To Constant  relop===  const=-1  OutDataTypeStr=boolean
  Data Store Read : DataStoreRead  DataStoreName=ArmIdPool  IndexOptions=Index vector (dialog)  Indices=1  OutputSizes=1
  Data Store Read1 : DataStoreRead  DataStoreName=FoundArm  IndexOptions=Index vector (dialog)  Indices=1  OutputSizes=1
  Data Store Read2 : DataStoreRead  DataStoreName=ArmIdPoolF  IndexOptions=Index vector (dialog)  Indices=1  OutputSizes=1
  Data Store Write1 : DataStoreWrite  DataStoreName=FoundArm  IndexOptions=Index vector (dialog)  Indices=1  OutputSizes=1
  Equal : RelationalOperator  Operator===  OutDataTypeStr=boolean  RndMeth=Simplest  InputSameDT=off
  For Iterator : ForIterator  IterationLimit=POOL_SIZE  IndexMode=Zero-based
  Selector : Selector  IndexMode=Zero-based  InputPortWidth=POOL_SIZE  IndexOptions=Index vector (port)  Indices=[1 3]  OutputSizes=1
  Selector1 : Selector  IndexMode=Zero-based  InputPortWidth=POOL_SIZE  IndexOptions=Index vector (port)  Indices=[1 3]  OutputSizes=1
  Switch : Switch  Criteria=u2 ~= 0  SaturateOnIntegerOverflow=off  InputSameDT=off
  Out1 : Outport
  wires:
  Data Store Read/1 -> Selector/1
  Selector/1 -> Equal/2
  Equal/1 -> AND1/1
  Switch/1 -> Data Store Write1/1, Out1/1
  Data Store Read1/1 -> Compare To Constant1/1, Switch/3
  Compare To Constant1/1 -> AND/2
  AND/1 -> Switch/2
  ArmId/1 -> Equal/1
  For Iterator/1 -> Selector1/2, Switch/1, Selector/2
  Selector1/1 -> Compare To Constant/1
  Data Store Read2/1 -> Selector1/1
  Compare To Constant/1 -> AND1/2
  AND1/1 -> AND/1

== system RAC/Main/Register/Handle/FindInPool/FindArmIdTInPool ==
  ArmId : Inport
  AND : Logic  IconShape=distinctive  AllPortsSameDT=off  OutDataTypeStr=boolean
  AND1 : Logic  IconShape=distinctive  AllPortsSameDT=off  OutDataTypeStr=boolean
  Compare To Constant : simulink/Logic and Bit Operations/Compare To Constant  relop===  const=1  OutDataTypeStr=boolean
  Compare To Constant1 : simulink/Logic and Bit Operations/Compare To Constant  relop===  const=-1  OutDataTypeStr=boolean
  Data Store Read : DataStoreRead  DataStoreName=ArmIdPool  IndexOptions=Index vector (dialog)  Indices=1  OutputSizes=1
  Data Store Read1 : DataStoreRead  DataStoreName=FoundArmT  IndexOptions=Index vector (dialog)  Indices=1  OutputSizes=1
  Data Store Read2 : DataStoreRead  DataStoreName=ArmIdPoolF  IndexOptions=Index vector (dialog)  Indices=1  OutputSizes=1
  Data Store Write1 : DataStoreWrite  DataStoreName=FoundArmT  IndexOptions=Index vector (dialog)  Indices=1  OutputSizes=1
  Equal : RelationalOperator  Operator===  OutDataTypeStr=boolean  RndMeth=Simplest  InputSameDT=off
  For Iterator : ForIterator  IterationLimit=POOL_SIZE  IndexMode=Zero-based
  Selector : Selector  IndexMode=Zero-based  InputPortWidth=POOL_SIZE  IndexOptions=Index vector (port)  Indices=[1 3]  OutputSizes=1
  Selector1 : Selector  IndexMode=Zero-based  InputPortWidth=POOL_SIZE  IndexOptions=Index vector (port)  Indices=[1 3]  OutputSizes=1
  Switch : Switch  Criteria=u2 ~= 0  SaturateOnIntegerOverflow=off  InputSameDT=off
  FindPT : Outport
  wires:
  Data Store Read/1 -> Selector/1
  Selector/1 -> Equal/2
  Equal/1 -> AND1/1
  Switch/1 -> Data Store Write1/1, FindPT/1
  Data Store Read1/1 -> Compare To Constant1/1, Switch/3
  Compare To Constant1/1 -> AND/2
  AND/1 -> Switch/2
  ArmId/1 -> Equal/1
  Compare To Constant/1 -> AND1/2
  Data Store Read2/1 -> Selector1/1
  For Iterator/1 -> Selector1/2, Switch/1, Selector/2
  Selector1/1 -> Compare To Constant/1
  AND1/1 -> AND/1

== system RAC/Main/Start/Handle/AddArmIdInPool/Register ==
  ArmId : Inport
  FindE : Inport  Port=2
  Assignment : Assignment  IndexMode=Zero-based  DiagnosticForDimensions=Warning  IndexOptions=Index vector (port)  Indices=1  OutputSizes=1
  Assignment1 : Assignment  IndexMode=Zero-based  DiagnosticForDimensions=Warning  IndexOptions=Index vector (port)  Indices=1  OutputSizes=1
  Constant : Constant  OutDataTypeStr=int32
  Data Store Read : DataStoreRead  DataStoreName=ArmIdPool  IndexOptions=Index vector (dialog)  Indices=1  OutputSizes=1
  Data Store Read1 : DataStoreRead  DataStoreName=ArmIdPoolF  IndexOptions=Index vector (dialog)  Indices=1  OutputSizes=1
  Data Store Write : DataStoreWrite  DataStoreName=ArmIdPool  IndexOptions=Index vector (dialog)  Indices=1  OutputSizes=1
  Data Store Write1 : DataStoreWrite  DataStoreName=ArmIdPoolF  IndexOptions=Index vector (dialog)  Indices=1  OutputSizes=1
  Equal : RelationalOperator  Operator===  OutDataTypeStr=boolean  RndMeth=Simplest  InputSameDT=off
  For Iterator : ForIterator  IterationLimit=POOL_SIZE  IndexMode=Zero-based
  Selector : Selector  IndexMode=Zero-based  InputPortWidth=POOL_SIZE  IndexOptions=Index vector (port)  Indices=[1 3]  OutputSizes=1
  Selector1 : Selector  IndexMode=Zero-based  InputPortWidth=POOL_SIZE  IndexOptions=Index vector (port)  Indices=[1 3]  OutputSizes=1
  Switch : Switch  Criteria=u2 > Threshold  SaturateOnIntegerOverflow=off  InputSameDT=off
  Switch1 : Switch  Criteria=u2 > Threshold  SaturateOnIntegerOverflow=off  InputSameDT=off
  wires:
  For Iterator/1 -> Assignment1/3, Selector1/2, Selector/2, Assignment/3, Equal/2
  Data Store Read/1 -> Assignment/1, Selector/1
  FindE/1 -> Equal/1
  Equal/1 -> Switch1/2, Switch/2
  ArmId/1 -> Switch/1
  Switch/1 -> Assignment/2
  Selector/1 -> Switch/3
  Assignment/1 -> Data Store Write/1
  Data Store Read1/1 -> Selector1/1, Assignment1/1
  Constant/1 -> Switch1/1
  Selector1/1 -> Switch1/3
  Switch1/1 -> Assignment1/2
  Assignment1/1 -> Data Store Write1/1

== system RAC/Main/Start/Handle/FindInPool/FindArmIdInPool ==
  ArmId : Inport
  AND : Logic  IconShape=distinctive  AllPortsSameDT=off  OutDataTypeStr=boolean
  Compare To Constant : simulink/Logic and Bit Operations/Compare To Constant  relop===  const=1  OutDataTypeStr=boolean
  Constant : Constant  OutDataTypeStr=int8
  Data Store Read : DataStoreRead  DataStoreName=ArmIdPool  IndexOptions=Index vector (dialog)  Indices=1  OutputSizes=1
  Data Store Read1 : DataStoreRead  DataStoreName=Found  IndexOptions=Index vector (dialog)  Indices=1  OutputSizes=1
  Data Store Read2 : DataStoreRead  DataStoreName=ArmIdPoolF  IndexOptions=Index vector (dialog)  Indices=1  OutputSizes=1
  Data Store Write1 : DataStoreWrite  DataStoreName=Found  IndexOptions=Index vector (dialog)  Indices=1  OutputSizes=1
  Equal : RelationalOperator  Operator===  OutDataTypeStr=boolean  RndMeth=Simplest  InputSameDT=off
  For Iterator : ForIterator  IterationLimit=POOL_SIZE  IndexMode=Zero-based
  Selector : Selector  IndexMode=Zero-based  InputPortWidth=POOL_SIZE  IndexOptions=Index vector (port)  Indices=[1 3]  OutputSizes=1
  Selector1 : Selector  IndexMode=Zero-based  InputPortWidth=POOL_SIZE  IndexOptions=Index vector (port)  Indices=[1 3]  OutputSizes=1
  Switch : Switch  Criteria=u2 ~= 0  SaturateOnIntegerOverflow=off  InputSameDT=off
  Out1 : Outport
  wires:
  For Iterator/1 -> Selector1/2, Selector/2
  Data Store Read/1 -> Selector/1
  Selector/1 -> Equal/1
  ArmId/1 -> Equal/2
  Equal/1 -> AND/1
  Constant/1 -> Switch/1
  Switch/1 -> Out1/1, Data Store Write1/1
  Data Store Read1/1 -> Switch/3
  Data Store Read2/1 -> Selector1/1
  Selector1/1 -> Compare To Constant/1
  Compare To Constant/1 -> AND/2
  AND/1 -> Switch/2
